simulink model "HybridStateChart"  (R2020a)
settings: Solver=FixedStepAuto  StartTime=0.0  StopTime=50  RelTol=1e-3  EnableMultiTasking=on
libraries: arduinolib x17, dspswit3 x1
settings Model: SimulationMode=external  SILPILModeSetting=veronly  ExtModeTrigDuration=2  Creator=Sarah Bassem  LastModifiedBy=Lord
settings DataIOCC: ReturnWorkspaceOutputs=off
settings OptimizationCC: EnhancedBackFolding=on  PassReuseOutputArgsAs=Individual arguments  ZeroExternalMemoryAtStartup=off  ZeroInternalMemoryAtStartup=off  MaxStackSize=64  OptimizeBlockOrder=speed  DifferentSizesBufferReuse=on  OptimizationCustomize=off  EfficientTunableParamExpr=on
settings DebuggingCC: ParameterTunabilityLossMsg=error  ArithmeticOperatorsInVariantConditions=warning
settings HardwareCC: ProdBitPerInt=16  ProdBitPerPointer=16  ProdBitPerSizeT=16  ProdBitPerPtrDiffT=16  ProdLargestAtomicFloat=None  ProdWordSize=8  ProdHWDeviceType=Atmel->AVR
settings SFSimCC: SimUseLocalCustomCode=off  MATLABDynamicMemAlloc=off  CustomCodeUndefinedFunction=UseInterfaceOnly
settings RTWCC: SystemTargetFile=ert.tlc  HardwareBoard=Arduino Mega 2560  TLCOptions=-aInlineSetEventsForThisBaseRateFcn=TLC_FALSE -aSuppressMultiTaskScheduler=TLC_FALSE -aRateBasedStepFcn=1  TemplateMakefile=ert_default_tmf  RTWUseLocalCustomCode=off  Toolchain=Arduino AVR  BuildConfiguration=Faster Runs
settings CodeAppCC: ForceParamTrailComments=on  IgnoreCustomStorageClasses=off  OperatorAnnotations=on  SimulinkDataObjDesc=on  SFDataObjDesc=on  InsertBlockDesc=on
settings ERTTargetCC: SupportContinuousTime=on  SupportVariableSizeSignals=on  ExtModeStaticAllocSize=2048

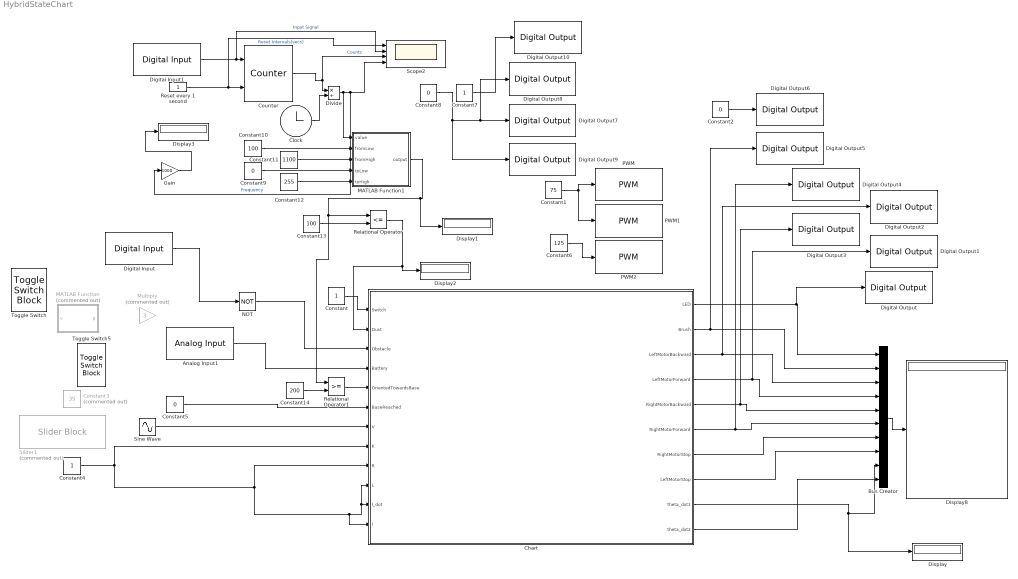
== system HybridStateChart ==
  Analog Input1 : arduinolib/Analog Input  pinNumber=6  ReadResultsOnly=off  ConversionTriggerSource=Software  ExternalTriggerType=uint32( 0 )  OutputDataType=uint16  EnableConversionCompleteNotify=off  EnableOuputStatus=off  SampleTime=-1  blockPlatform=arduino
  Bus Creator : BusCreator  Inputs=10
  Chart : Stateflow chart  TreatAsAtomicUnit=on
  Clock : Clock
  Constant : Constant
  Constant1 : Constant  Value=75
  Constant10 : Constant  Value=100
  Constant11 : Constant  Value=1100
  Constant12 : Constant  Value=255
  Constant13 : Constant  Value=100
  Constant14 : Constant  Value=200
  Constant{2,5,8..9} (4 alike) : Constant  Value=0
  Constant3 : Constant  Commented=on  Value=35
  Constant4 : Constant
  Constant6 : Constant  Value=125
  Constant7 : Constant
  Counter : dspswit3/Counter  Direction=Up  CountEvent=Rising edge  CounterSize=User defined  MaxCount=12000  InitialCount=0  Output=Count  HitValue=1  ResetInput=on  SamplesPerFrame=1  Ts=1  CntDtype=double  HitDtype=Logical
  Digital Input : arduinolib/Digital Input  pinNumber=4  Direction=input  SampleTime=0.1  blockPlatform=arduino
  Digital Input1 : arduinolib/Digital Input  pinNumber=19  Direction=input  SampleTime=0.1  blockPlatform=arduino
  Digital Output : arduinolib/Digital Output  pinNumber=18  Direction=output  blockPlatform=arduino
  Digital Output1 : arduinolib/Digital Output  pinNumber=3  Direction=output  blockPlatform=arduino
  Digital Output10 : arduinolib/Digital Output  pinNumber=14  Direction=output  blockPlatform=arduino
  Digital Output2 : arduinolib/Digital Output  pinNumber=2  Direction=output  blockPlatform=arduino
  Digital Output3 : arduinolib/Digital Output  pinNumber=8  Direction=output  blockPlatform=arduino
  Digital Output4 : arduinolib/Digital Output  pinNumber=7  Direction=output  blockPlatform=arduino
  Digital Output5 : arduinolib/Digital Output  pinNumber=12  Direction=output  blockPlatform=arduino
  Digital Output6 : arduinolib/Digital Output  pinNumber=11  Direction=output  blockPlatform=arduino
  Digital Output7 : arduinolib/Digital Output  pinNumber=16  Direction=output  blockPlatform=arduino
  Digital Output8 : arduinolib/Digital Output  pinNumber=15  Direction=output  blockPlatform=arduino
  Digital Output9 : arduinolib/Digital Output  pinNumber=17  Direction=output  blockPlatform=arduino
  Display{,1..3,8} (5 alike) : Display
  Divide : Product  Inputs=*/
  Gain : Gain  Gain=1000
  MATLAB Function : MATLAB Function  Commented=on  TreatAsAtomicUnit=on
  MATLAB Function1 : MATLAB Function  TreatAsAtomicUnit=on
  Multiply : Gain  Commented=on  Gain=3
  NOT : Logic  Operator=NOT  IconShape=distinctive  AllPortsSameDT=off  OutDataTypeStr=boolean
  PWM : arduinolib/PWM  pinNumber=9  frequencyType=Default  desiredFrequency=490.2  achievableFrequency=490.2
  PWM1 : arduinolib/PWM  pinNumber=6  frequencyType=Default  desiredFrequency=490.2  achievableFrequency=490.2
  PWM2 : arduinolib/PWM  pinNumber=13  frequencyType=Default  desiredFrequency=490.2  achievableFrequency=490.2
  Relational Operator : RelationalOperator  Operator=<=  OutDataTypeStr=boolean  RndMeth=Simplest
  Relational Operator1 : RelationalOperator  OutDataTypeStr=boolean  RndMeth=Simplest
  Reset every 1 second : Constant
  Scope2 : Scope  NumInputPorts=4
  Sine Wave : Sin  SampleTime=0
  Slider1 : SliderBlock  Commented=on
  Toggle Switch : ToggleSwitchBlock
      settings: Values={{'Off', 'On'}, [0 1]}
  Toggle Switch5 : ToggleSwitchBlock
      settings: Values={{'Off', 'On'}, [0 1]}
  wires:
  Constant/1 -> Chart/1(Switch)
  Digital Input/1 -> NOT/1
  Constant5/1 -> Chart/6(BaseReached)
  Bus Creator/1 -> Display8/1
  Chart/1(LED) -> Digital Output/1, Bus Creator/1
  Chart/2(Brush) -> Digital Output5/1, Bus Creator/2
  Chart/3(LeftMotorBackward) -> Digital Output2/1, Bus Creator/3
  Chart/4(LeftMotorForward) -> Digital Output1/1, Bus Creator/4
  Chart/5(RightMotorBackward) -> Digital Output3/1, Bus Creator/5
  Chart/6(RightMotorForward) -> Digital Output4/1, Bus Creator/6
  Chart/7(RightMotorStop) -> Bus Creator/7
  Chart/8(LeftMotorStop) -> Bus Creator/8
  Constant4/1 -> Chart/12(I), Chart/11(I_dot), Chart/10(L), Chart/9(R), Chart/8(K)
  Chart/9(theta_dot1) -> Display/1, Bus Creator/9
  Chart/10(theta_dot2) -> Bus Creator/10
  Sine Wave/1 -> Chart/7(V)
  Constant1/1 -> PWM1/1, PWM/1
  Constant2/1 -> Digital Output6/1
  Analog Input1/1 -> Chart/4(Battery)
  NOT/1 -> Chart/3(Obstacle)
  Constant6/1 -> PWM2/1
  Clock/1 -> Divide/2
  Counter/1 -> Scope2/3, Divide/1  "Counts"
  Reset every 1 second/1 -> Scope2/1, Counter/2  "Reset Intervals(secs)"
  Digital Input1/1 -> Counter/1, Scope2/2  "Input Signal"
  Divide/1 -> Gain/1, Scope2/4, MATLAB Function1/1(value)  "Frequency"
  Constant7/1 -> Digital Output10/1
  Constant8/1 -> Digital Output8/1, Digital Output7/1, Digital Output9/1
  Constant9/1 -> MATLAB Function1/4(toLow)
  Constant10/1 -> MATLAB Function1/2(fromLow)
  Constant11/1 -> MATLAB Function1/3(fromHigh)
  Constant12/1 -> MATLAB Function1/5(toHigh)
  MATLAB Function1/1(output) -> Display1/1, Relational Operator1/1, Relational Operator/1
  Constant13/1 -> Relational Operator/2
  Relational Operator1/1 -> Chart/5(OrientedTowardsBase)
  Constant14/1 -> Relational Operator1/2
  Relational Operator/1 -> Display2/1, Chart/2(Dust)
  Gain/1 -> Display3/1

== matlab function HybridStateChart/MATLAB Function ==
  data: v input; p output
function p  = BatteryVolt(v)
if v<9
    p=100;
else
    x = [10.5 11.31 11.58 11.75 11.9 12.06 12.20 12.32 12.42 12.5 12.7];
    y = [0 10 20 30 40 50 60 70 80 90 100];
%     p = polyfit(x,y,0);
%     y1 = polyval(p,x);
%     %pchip() - Hermitian
%     xx = x;

    p=pchip(x,y,v);
end
end

== stateflow chart HybridStateChart/Chart ==
  settings: updateMethod=CONTINUOUS
  state Ground_Cleaning_Robot
    (history)
    state Robot_OFF
      during: Brush=0;
      LeftMotorStop=1; RightMotorStop=1; RightMotorForward=0;RightMotorBackward=0;LeftMotorForward=0;LeftMotorBackward=0;LED=0;
    state Robot_ON
      state Movement [parallel]
        settings: executionOrder=1
        (history)
        state Stop
          during: theta_dot1=(V-L*I_dot-R*I)/K;
          theta_dot2=(V-L*I_dot-R*I)/K;
          during: LeftMotorStop=1;
          RightMotorStop=1;
          LeftMotorForward=0;
          LeftMotorBackward=0;
          RightMotorForward=0;
          RightMotorBackward=0;
        state Forward
          during: theta_dot1=(V-L*I_dot-R*I)/K;
          theta_dot2=(V-L*I_dot-R*I)/K;
          entry: BackTimer=0;
          during: LeftMotorForward=1;
          RightMotorForward=1;
          LeftMotorBackward=0; RightMotorBackward=0;
          LeftMotorStop=0; RightMotorStop=0;
        state Backward
          during: theta_dot1=(V-L*I_dot-R*I)/K;
          theta_dot2=(V-L*I_dot-R*I)/K;
          entry: RotateTimer=0;
          during: LeftMotorBackward=1;
          RightMotorBackward=1;
          LeftMotorForward=0; RightMotorForward=0;
          LeftMotorStop=0;RightMotorStop=0;
        state Rotate
          during: theta_dot1=(V-L*I_dot-R*I)/K;
          theta_dot2=0;
          during: LeftMotorBackward=1;
          RightMotorForward=1;
          LeftMotorStop=0; RightMotorStop=0;
          LeftMotorForward=0; RightMotorBackward=0;
        Stop -> Backward [order 2] : [Battery==100]
        Forward -> Stop [order 2] : [BaseReached==1 && Battery<20]
        (default) -> Forward
        Rotate -> Forward [order 1] : [after(1,sec) && Obstacle==0]
        Forward -> Rotate [order 3] : [Battery<20]{LED=1;}
        Rotate -> Forward [order 2] : [OrientedTowardsBase==1]
        Forward -> Backward [order 1] : [Obstacle==1]
        Backward -> Backward [order 2] : [Obstacle==1]
        Backward -> Rotate [order 1] : [after(1,sec) && Obstacle==0]
      state Cleaning [parallel]
        settings: executionOrder=2
        (history)
        state OFF
          during: Brush=0;
        state ON
          during: Brush=1;
        Ground_Cleaning_Robot.Robot_ON.Cleaning.OFF -> Ground_Cleaning_Robot.Robot_ON.Cleaning.ON : [Dust==1 && Battery>20]
        Ground_Cleaning_Robot.Robot_ON.Cleaning.ON -> Ground_Cleaning_Robot.Robot_ON.Cleaning.OFF : [Dust==0]
      state Charging [parallel]
        settings: executionOrder=3
        (history)
        state OFF
          entry: LED=0;
        state ON
          entry: LED=1;
        (default) -> Ground_Cleaning_Robot.Robot_ON.Charging.OFF
        Ground_Cleaning_Robot.Robot_ON.Charging.ON -> Ground_Cleaning_Robot.Robot_ON.Charging.OFF : [Battery==100]
      (default) -> Ground_Cleaning_Robot.Robot_ON.Cleaning.OFF
      Stop -> Ground_Cleaning_Robot.Robot_ON.Charging.ON [order 1] : [BaseReached==1 && Battery<20]
    Robot_OFF -> Robot_ON : [Switch==1]
    Robot_ON -> Robot_OFF : [Switch==0]
  (default) -> Robot_OFF
  data: Switch input; LED output; Brush output; Dust input; LeftMotorBackward output; LeftMotorForward output; RightMotorBackward output; RightMotorForward output; RightMotorStop output; Obstacle input; Battery input; OrientedTowardsBase input; BaseReached input; BackTimer local; RotateTimer local; LeftMotorStop output; V input; K input; R input; L input; theta_dot1 output; theta_dot2 output; I_dot input; I input

== matlab function HybridStateChart/MATLAB Function1 ==
  data: value input; output output; fromLow input; fromHigh input; toLow input; toHigh input
function output = mapfun(value,fromLow,fromHigh,toLow,toHigh)
narginchk(5,5)
nargoutchk(0,1)
output = (value - fromLow) .* (toHigh - toLow) ./ (fromHigh - fromLow) + toLow;
end
